simulink model "prob3"  (R2020b)
settings: Solver=VariableStepAuto  StartTime=0.0  StopTime=10.0  RelTol=1e-3
values from neighbouring files (symbols this model uses):
  b = 50.0    [PI_controller_data.sldd]
  ki = 30.0    [PI_controller_data.sldd]
  kp = 700.0    [PI_controller_data.sldd]
  M = 1000.0    [PI_controller_data.sldd]
settings Model: Creator=DELL  LastModifiedBy=DELL

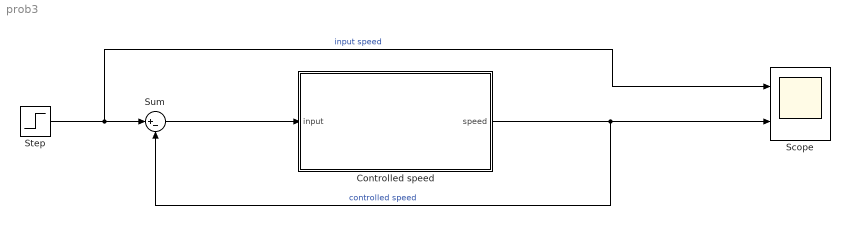
== system prob3 ==
  Controlled speed : Subsystem  TreatAsAtomicUnit=on
  Scope : Scope  NumInputPorts=2
  Step : Step  Time=0  After=u  SampleTime=0
  Sum : Sum  Inputs=|+-
  wires:
  Controlled speed/1(speed) -> Scope/2, Sum/2  "controlled speed"
  Step/1 -> Scope/1, Sum/1  "input speed"
  Sum/1 -> Controlled speed/1(input)

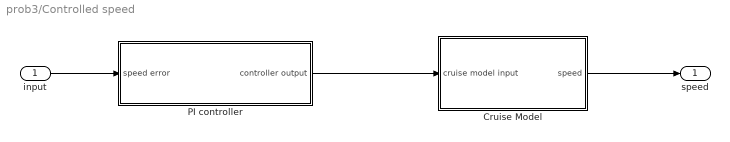
== system prob3/Controlled speed ==
  input : Inport
  Cruise Model : Subsystem
  PI controller : Subsystem
  speed : Outport
  wires:
  PI controller/1(controller output) -> Cruise Model/1(cruise model input)
  input/1 -> PI controller/1(speed error)
  Cruise Model/1(speed) -> speed/1

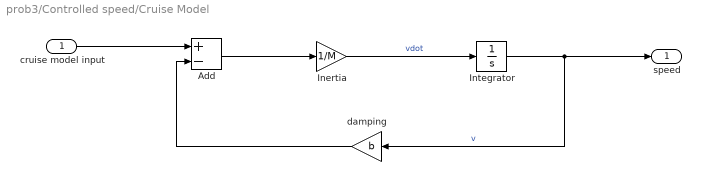
== system prob3/Controlled speed/Cruise Model ==
  cruise model input : Inport
  Add : Sum  Inputs=+-
  Inertia : Gain  Gain=1/M
  Integrator : Integrator
  damping : Gain  Gain=b
  speed : Outport
  wires:
  Integrator/1 -> speed/1, damping/1  "v"
  damping/1 -> Add/2
  cruise model input/1 -> Add/1
  Inertia/1 -> Integrator/1  "vdot"
  Add/1 -> Inertia/1

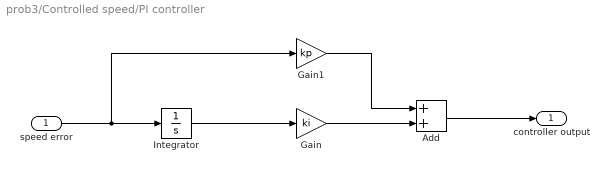
== system prob3/Controlled speed/PI controller ==
  speed error : Inport
  Add : Sum
  Gain : Gain  Gain=ki
  Gain1 : Gain  Gain=kp
  Integrator : Integrator
  controller output : Outport
  wires:
  Gain/1 -> Add/2
  Integrator/1 -> Gain/1
  Gain1/1 -> Add/1
  Add/1 -> controller output/1
  speed error/1 -> Gain1/1, Integrator/1
